simulink model "DDCU_wxt_v02_forA_OpenLoop"  (R2014a)
settings: Solver=FixedStepDiscrete  StartTime=0.0  StopTime=16  FixedStep=0.05  RelTol=1e-3
InitFcn:
  | Veh_Par_wxt
values from neighbouring files (symbols this model uses):
  ag_thr = 0.4*g    (= 3.924)    [Veh_Par_wxt.m]
  B = 2.25    [Veh_Par_wxt.m]
  bra_pre_em = 12    [Veh_Par_wxt.m]
  bra_pre_gz2 = 12/3    (= 4)    [Veh_Par_wxt.m]
  bra_pre_gz34 = 12/3    (= 4)    [Veh_Par_wxt.m]
  bra_pre_yd = 12/2    (= 6)    [Veh_Par_wxt.m]
  brakepre_dem_data = [0 1 2 3 4 5 6 7 8 9 10 11 12]    [Veh_Par_wxt.m]
  brakeTrq_dem_data = [0 218.198 436.396 654.594 872.792 1090.99 1309.188 1527.386 1745.584 1963.782 2181.98 2400.178 2618.376]    [Veh_Par_wxt.m]
  bratrq_max = 4*2618.376    (= 10473.504)    [Veh_Par_wxt.m]
  eff_tran = 0.75    [Veh_Par_wxt.m]
  G = Mass*g    (= 36297)    [Veh_Par_wxt.m]
  kd1 = 1    [Veh_Par_wxt.m]
  kd2 = 1    [Veh_Par_wxt.m]
  kd3 = 1    [Veh_Par_wxt.m]
  ki1 = 1    [Veh_Par_wxt.m]
  ki2 = 1    [Veh_Par_wxt.m]
  ki3 = 1    [Veh_Par_wxt.m]
  kp1 = 1    [Veh_Par_wxt.m]
  kp2 = 1    [Veh_Par_wxt.m]
  kp3 = 1    [Veh_Par_wxt.m]
  L = 3.12    [Veh_Par_wxt.m]
  premax = 12    [Veh_Par_wxt.m]
  Radius = 0.20    (= 0.2)    [Veh_Par_wxt.m]
  s_opt_yi_add = 0.05    [Veh_Par_wxt.m]
  s_opt_zhuan_add = 0.05    [Veh_Par_wxt.m]
  spd_map_mot = [0 100 200 300 360 400 500 600 700 800 900]*tras_ratio    [Veh_Par_wxt.m]
  spdmax = 900*tras_ratio    (= 5580)    [Veh_Par_wxt.m]
  speed_thr_park = 5/3.6/Radius*30/pi    (= 66.3145596216)    [Veh_Par_wxt.m]
  tras_ratio = 6.2    [Veh_Par_wxt.m]
  trq_map_mot = [1200 1200 1200 1200 1200 1080 864 720 617 540 480]/tras_ratio    [Veh_Par_wxt.m]
  trqmax = 80    [Veh_Par_wxt.m]
  v_thr1_b = 5    [Veh_Par_wxt.m]
  v_thr2_b = 20    [Veh_Par_wxt.m]
  v_thr_park = 5    [Veh_Par_wxt.m]
undefined symbols (not defined in the file or in its folder): DiscIntNeverNeededParam, sigbuilder_block
libraries: simulink x169, ec5744lib x9
(part 5 of 13)

== system DDCU_wxt_v02_forA_OpenLoop/OutputSignalProcess/VCU_MCU2_replace/M4Mode ==
  M4Mode : Inport
  Constant{1..4,6..8} (7 alike) : Constant  Value=0  OutDataTypeStr=uint8
  M4ModeRon : Rounding  Operator=round
  M4Mode_1sat : Saturate  UpperLimit=3  LowerLimit=0
  M4Mode_Convert : DataTypeConversion  OutDataTypeStr=uint8
  M4Mode_Convert1 : DataTypeConversion  OutDataTypeStr=uint32
  M4Mode_D : Product  Inputs=*/
  M4Mode_F : Constant  OutDataTypeStr=single
  M4Mode_L : simulink/Logic and Bit Operations/Bitwise Operator  logicop=AND  UseBitMask=on  BitMask=3  BitMaskRealWorld=Stored Integer
  M4Mode_O : Constant  Value=0  OutDataTypeStr=single
  M4Mode_S : ArithShift
  M4Mode_sat : Saturate  UpperLimit=3  LowerLimit=0
  M4Mode_st : Sum  Inputs=+-
  output1 : Outport
  output2 : Outport  Port=2
  output3 : Outport  Port=3
  output4 : Outport  Port=4
  output5 : Outport  Port=5
  output6 : Outport  Port=6
  output7 : Outport  Port=7
  output8 : Outport  Port=8
  wires:
  M4Mode/1 -> M4Mode_sat/1
  M4Mode_sat/1 -> M4Mode_st/1
  M4Mode_O/1 -> M4Mode_st/2
  M4Mode_st/1 -> M4Mode_D/1
  M4Mode_F/1 -> M4Mode_D/2
  M4Mode_D/1 -> M4ModeRon/1
  M4ModeRon/1 -> M4Mode_S/1
  M4Mode_S/1 -> M4Mode_1sat/1
  M4Mode_1sat/1 -> M4Mode_Convert1/1
  M4Mode_Convert1/1 -> M4Mode_L/1
  M4Mode_L/1 -> M4Mode_Convert/1
  M4Mode_Convert/1 -> output5/1
  Constant1/1 -> output1/1
  Constant2/1 -> output2/1
  Constant3/1 -> output3/1
  Constant4/1 -> output4/1
  Constant6/1 -> output6/1
  Constant7/1 -> output7/1
  Constant8/1 -> output8/1

== system DDCU_wxt_v02_forA_OpenLoop/OutputSignalProcess/VCU_MCU2_replace/M4SpeedLimit ==
  M4SpeedLimit : Inport
  Constant{1..6} (6 alike) : Constant  Value=0  OutDataTypeStr=uint8
  M4SpeedLimitBitCov : DataTypeConversion  OutDataTypeStr=uint8
  M4SpeedLimitCOV : DataTypeConversion  OutDataTypeStr=uint8
  M4SpeedLimitRon : Rounding  Operator=round
  M4SpeedLimit_1sat : Saturate  UpperLimit=4095  LowerLimit=0
  M4SpeedLimit_And : simulink/Logic and Bit Operations/Bitwise Operator  logicop=AND  UseBitMask=off  NumInputPorts=2  BitMask=bin2dec('11011001')  BitMaskRealWorld=Stored Integer
  M4SpeedLimit_And_C : Constant  Value=255  OutDataTypeStr=uint32
  M4SpeedLimit_Convert : DataTypeConversion  OutDataTypeStr=uint32
  M4SpeedLimit_D : Product  Inputs=*/
  M4SpeedLimit_D1 : Product  Inputs=*/
  M4SpeedLimit_F : Constant  Value=5  OutDataTypeStr=single
  M4SpeedLimit_L : simulink/Logic and Bit Operations/Bitwise Operator  logicop=AND  UseBitMask=on  BitMask=4095  BitMaskRealWorld=Stored Integer
  M4SpeedLimit_O : Constant  Value=0  OutDataTypeStr=single
  M4SpeedLimit_S : ArithShift
  M4SpeedLimit_sat : Saturate  UpperLimit=20475  LowerLimit=0
  M4SpeedLimit_st : Sum  Inputs=+-
  M4SpeedLimitoutput8_C : Constant  Value=256
  output1 : Outport
  output2 : Outport  Port=2
  output3 : Outport  Port=3
  output4 : Outport  Port=4
  output5 : Outport  Port=5
  output6 : Outport  Port=6
  output7 : Outport  Port=7
  output8 : Outport  Port=8
  wires:
  M4SpeedLimit/1 -> M4SpeedLimit_sat/1
  M4SpeedLimit_sat/1 -> M4SpeedLimit_st/1
  M4SpeedLimit_O/1 -> M4SpeedLimit_st/2
  M4SpeedLimit_st/1 -> M4SpeedLimit_D/1
  M4SpeedLimit_F/1 -> M4SpeedLimit_D/2
  M4SpeedLimit_D/1 -> M4SpeedLimitRon/1
  M4SpeedLimitRon/1 -> M4SpeedLimit_S/1
  M4SpeedLimit_S/1 -> M4SpeedLimit_1sat/1
  M4SpeedLimit_1sat/1 -> M4SpeedLimit_Convert/1
  M4SpeedLimit_Convert/1 -> M4SpeedLimit_L/1
  M4SpeedLimit_L/1 -> M4SpeedLimit_D1/1, M4SpeedLimit_And/1
  M4SpeedLimitoutput8_C/1 -> M4SpeedLimit_D1/2
  M4SpeedLimit_D1/1 -> M4SpeedLimitCOV/1
  M4SpeedLimitCOV/1 -> output8/1
  M4SpeedLimit_And_C/1 -> M4SpeedLimit_And/2
  M4SpeedLimit_And/1 -> M4SpeedLimitBitCov/1
  M4SpeedLimitBitCov/1 -> output7/1
  Constant1/1 -> output1/1
  Constant2/1 -> output2/1
  Constant3/1 -> output3/1
  Constant4/1 -> output4/1
  Constant5/1 -> output5/1
  Constant6/1 -> output6/1

== system DDCU_wxt_v02_forA_OpenLoop/OutputSignalProcess/VCU_MCU2_replace/M4SpeedSet ==
  M4SpeedSet : Inport
  Constant{1..4,7..8} (6 alike) : Constant  Value=0  OutDataTypeStr=uint8
  M4SpeedSetBitCov : DataTypeConversion  OutDataTypeStr=uint8
  M4SpeedSetCOV : DataTypeConversion  OutDataTypeStr=uint8
  M4SpeedSetRon : Rounding  Operator=round
  M4SpeedSet_1sat : Saturate  UpperLimit=65520  LowerLimit=0
  M4SpeedSet_And : simulink/Logic and Bit Operations/Bitwise Operator  logicop=AND  UseBitMask=off  NumInputPorts=2  BitMask=bin2dec('11011001')  BitMaskRealWorld=Stored Integer
  M4SpeedSet_And_C : Constant  Value=255  OutDataTypeStr=uint32
  M4SpeedSet_Convert : DataTypeConversion  OutDataTypeStr=uint32
  M4SpeedSet_D : Product  Inputs=*/
  M4SpeedSet_D1 : Product  Inputs=*/
  M4SpeedSet_F : Constant  Value=5  OutDataTypeStr=single
  M4SpeedSet_L : simulink/Logic and Bit Operations/Bitwise Operator  logicop=AND  UseBitMask=on  BitMask=65520  BitMaskRealWorld=Stored Integer
  M4SpeedSet_O : Constant  Value=-5000  OutDataTypeStr=single
  M4SpeedSet_S : ArithShift  BitShiftNumber=-4
  M4SpeedSet_sat : Saturate  UpperLimit=15475  LowerLimit=-5000
  M4SpeedSet_st : Sum  Inputs=+-
  M4SpeedSetoutput6_C : Constant  Value=256
  output1 : Outport
  output2 : Outport  Port=2
  output3 : Outport  Port=3
  output4 : Outport  Port=4
  output5 : Outport  Port=5
  output6 : Outport  Port=6
  output7 : Outport  Port=7
  output8 : Outport  Port=8
  wires:
  M4SpeedSet/1 -> M4SpeedSet_sat/1
  M4SpeedSet_sat/1 -> M4SpeedSet_st/1
  M4SpeedSet_O/1 -> M4SpeedSet_st/2
  M4SpeedSet_st/1 -> M4SpeedSet_D/1
  M4SpeedSet_F/1 -> M4SpeedSet_D/2
  M4SpeedSet_D/1 -> M4SpeedSetRon/1
  M4SpeedSetRon/1 -> M4SpeedSet_S/1
  M4SpeedSet_S/1 -> M4SpeedSet_1sat/1
  M4SpeedSet_1sat/1 -> M4SpeedSet_Convert/1
  M4SpeedSet_Convert/1 -> M4SpeedSet_L/1
  M4SpeedSet_L/1 -> M4SpeedSet_D1/1, M4SpeedSet_And/1
  M4SpeedSetoutput6_C/1 -> M4SpeedSet_D1/2
  M4SpeedSet_D1/1 -> M4SpeedSetCOV/1
  M4SpeedSetCOV/1 -> output6/1
  M4SpeedSet_And_C/1 -> M4SpeedSet_And/2
  M4SpeedSet_And/1 -> M4SpeedSetBitCov/1
  M4SpeedSetBitCov/1 -> output5/1
  Constant1/1 -> output1/1
  Constant2/1 -> output2/1
  Constant3/1 -> output3/1
  Constant4/1 -> output4/1
  Constant7/1 -> output7/1
  Constant8/1 -> output8/1

== system DDCU_wxt_v02_forA_OpenLoop/OutputSignalProcess/VCU_MCU2_replace/MCU2HeartBeat ==
  MCU2HeartBeat : Inport
  Constant{1..7} (7 alike) : Constant  Value=0  OutDataTypeStr=uint8
  MCU2HeartBeatRon : Rounding  Operator=round
  MCU2HeartBeat_1sat : Saturate  UpperLimit=240  LowerLimit=0
  MCU2HeartBeat_Convert : DataTypeConversion  OutDataTypeStr=uint8
  MCU2HeartBeat_Convert1 : DataTypeConversion  OutDataTypeStr=uint32
  MCU2HeartBeat_D : Product  Inputs=*/
  MCU2HeartBeat_F : Constant  OutDataTypeStr=single
  MCU2HeartBeat_L : simulink/Logic and Bit Operations/Bitwise Operator  logicop=AND  UseBitMask=on  BitMask=240  BitMaskRealWorld=Stored Integer
  MCU2HeartBeat_O : Constant  Value=0  OutDataTypeStr=single
  MCU2HeartBeat_S : ArithShift  BitShiftNumber=-4
  MCU2HeartBeat_sat : Saturate  UpperLimit=15  LowerLimit=0
  MCU2HeartBeat_st : Sum  Inputs=+-
  output1 : Outport
  output2 : Outport  Port=2
  output3 : Outport  Port=3
  output4 : Outport  Port=4
  output5 : Outport  Port=5
  output6 : Outport  Port=6
  output7 : Outport  Port=7
  output8 : Outport  Port=8
  wires:
  MCU2HeartBeat/1 -> MCU2HeartBeat_sat/1
  MCU2HeartBeat_sat/1 -> MCU2HeartBeat_st/1
  MCU2HeartBeat_O/1 -> MCU2HeartBeat_st/2
  MCU2HeartBeat_st/1 -> MCU2HeartBeat_D/1
  MCU2HeartBeat_F/1 -> MCU2HeartBeat_D/2
  MCU2HeartBeat_D/1 -> MCU2HeartBeatRon/1
  MCU2HeartBeatRon/1 -> MCU2HeartBeat_S/1
  MCU2HeartBeat_S/1 -> MCU2HeartBeat_1sat/1
  MCU2HeartBeat_1sat/1 -> MCU2HeartBeat_Convert1/1
  MCU2HeartBeat_Convert1/1 -> MCU2HeartBeat_L/1
  MCU2HeartBeat_L/1 -> MCU2HeartBeat_Convert/1
  MCU2HeartBeat_Convert/1 -> output8/1
  Constant1/1 -> output1/1
  Constant2/1 -> output2/1
  Constant3/1 -> output3/1
  Constant4/1 -> output4/1
  Constant5/1 -> output5/1
  Constant6/1 -> output6/1
  Constant7/1 -> output7/1

== system DDCU_wxt_v02_forA_OpenLoop/OutputSignalProcess/VCU_Park/ParkEnable ==
  ParkEnable : Inport
  Constant{2..8} (7 alike) : Constant  Value=0  OutDataTypeStr=uint8
  ParkEnableRon : Rounding  Operator=round
  ParkEnable_1sat : Saturate  UpperLimit=1  LowerLimit=0
  ParkEnable_Convert : DataTypeConversion  OutDataTypeStr=uint8
  ParkEnable_Convert1 : DataTypeConversion  OutDataTypeStr=uint32
  ParkEnable_D : Product  Inputs=*/
  ParkEnable_F : Constant  OutDataTypeStr=single
  ParkEnable_L : simulink/Logic and Bit Operations/Bitwise Operator  logicop=AND  UseBitMask=on  BitMask=1  BitMaskRealWorld=Stored Integer
  ParkEnable_O : Constant  Value=0  OutDataTypeStr=single
  ParkEnable_S : ArithShift
  ParkEnable_sat : Saturate  UpperLimit=1  LowerLimit=0
  ParkEnable_st : Sum  Inputs=+-
  output1 : Outport
  output2 : Outport  Port=2
  output3 : Outport  Port=3
  output4 : Outport  Port=4
  output5 : Outport  Port=5
  output6 : Outport  Port=6
  output7 : Outport  Port=7
  output8 : Outport  Port=8
  wires:
  ParkEnable/1 -> ParkEnable_sat/1
  ParkEnable_sat/1 -> ParkEnable_st/1
  ParkEnable_O/1 -> ParkEnable_st/2
  ParkEnable_st/1 -> ParkEnable_D/1
  ParkEnable_F/1 -> ParkEnable_D/2
  ParkEnable_D/1 -> ParkEnableRon/1
  ParkEnableRon/1 -> ParkEnable_S/1
  ParkEnable_S/1 -> ParkEnable_1sat/1
  ParkEnable_1sat/1 -> ParkEnable_Convert1/1
  ParkEnable_Convert1/1 -> ParkEnable_L/1
  ParkEnable_L/1 -> ParkEnable_Convert/1
  ParkEnable_Convert/1 -> output1/1
  Constant2/1 -> output2/1
  Constant3/1 -> output3/1
  Constant4/1 -> output4/1
  Constant5/1 -> output5/1
  Constant6/1 -> output6/1
  Constant7/1 -> output7/1
  Constant8/1 -> output8/1

== system DDCU_wxt_v02_forA_OpenLoop/Data_Input/HCU1_VCU/HCU1_VCU/acc_Sub ==
  In1 : Inport
  Out1 : Outport
  wires:
  In1/1 -> Out1/1

== system DDCU_wxt_v02_forA_OpenLoop/Data_Input/HCU1_VCU/HCU1_VCU/break_Sub ==
  In1 : Inport
  Out1 : Outport
  wires:
  In1/1 -> Out1/1

== system DDCU_wxt_v02_forA_OpenLoop/Data_Input/HCU1_VCU/HCU1_VCU/pwr_limit_Sub ==
  In1 : Inport
  Out1 : Outport
  wires:
  In1/1 -> Out1/1

== system DDCU_wxt_v02_forA_OpenLoop/Data_Input/HCU1_VCU/HCU1_VCU/real_velocity_Sub ==
  In1 : Inport
  Out1 : Outport
  wires:
  In1/1 -> Out1/1

== system DDCU_wxt_v02_forA_OpenLoop/Data_Input/HCU1_VCU/HCU1_VCU/turn_Sub ==
  In1 : Inport
  Out1 : Outport
  wires:
  In1/1 -> Out1/1

== system DDCU_wxt_v02_forA_OpenLoop/Data_Input/HCU1_VCU1/MUC1_VCU1/spd_mot_lf_Sub ==
  In1 : Inport
  Out1 : Outport
  wires:
  In1/1 -> Out1/1

== system DDCU_wxt_v02_forA_OpenLoop/Data_Input/HCU1_VCU1/MUC1_VCU1/spd_mot_lr_Sub ==
  In1 : Inport
  Out1 : Outport
  wires:
  In1/1 -> Out1/1

== system DDCU_wxt_v02_forA_OpenLoop/Data_Input/HCU1_VCU1/MUC1_VCU1/spd_mot_rf_Sub ==
  In1 : Inport
  Out1 : Outport
  wires:
  In1/1 -> Out1/1

== system DDCU_wxt_v02_forA_OpenLoop/Data_Input/HCU1_VCU1/MUC1_VCU1/spd_mot_rr_Sub ==
  In1 : Inport
  Out1 : Outport
  wires:
  In1/1 -> Out1/1

== system DDCU_wxt_v02_forA_OpenLoop/Data_Input/HCU2_VCU/HCU2_VCU/daodang_Sub ==
  In1 : Inport
  Out1 : Outport
  wires:
  In1/1 -> Out1/1

== system DDCU_wxt_v02_forA_OpenLoop/Data_Input/HCU2_VCU/HCU2_VCU/kongdang_Sub ==
  In1 : Inport
  Out1 : Outport
  wires:
  In1/1 -> Out1/1

== system DDCU_wxt_v02_forA_OpenLoop/Data_Input/HCU2_VCU/HCU2_VCU/qianjin_Sub ==
  In1 : Inport
  Out1 : Outport
  wires:
  In1/1 -> Out1/1

== system DDCU_wxt_v02_forA_OpenLoop/Data_Input/HCU2_VCU/HCU2_VCU/zhongxinzhuanxiang_Sub ==
  In1 : Inport
  Out1 : Outport
  wires:
  In1/1 -> Out1/1

== system DDCU_wxt_v02_forA_OpenLoop/Data_Input/HCU2_VCU/HCU2_VCU/zhuche_Sub ==
  In1 : Inport
  Out1 : Outport
  wires:
  In1/1 -> Out1/1

== system DDCU_wxt_v02_forA_OpenLoop/MainControl/mode_control/Park/park ==
  Signals : Inport
  1-D Lookup Table : Lookup_n-D  NumberOfTableDimensions=1  BreakpointsForDimension1=brakeTrq_dem_data  Table=brakepre_dem_data  InternalRulePriority=Speed  RndMeth=Simplest  InputSameDT=on
  1-D Lookup Table1 : Lookup_n-D  NumberOfTableDimensions=1  BreakpointsForDimension1=brakeTrq_dem_data  Table=brakepre_dem_data  InternalRulePriority=Speed  RndMeth=Simplest  InputSameDT=on
  Bus Selector : BusSelector  OutputSignals=YaoKong.brake_dem
  Constant : Constant  Value=bratrq_max
  Gain : Gain  Gain=1/2
  Gain1 : Gain  Gain=1/100
  Gain2 : Gain  Gain=1/2
  Gain3 : Gain  Gain=1/2
  HeartBeat : MATLAB Function  TreatAsAtomicUnit=on
  HeartBeat1 : MATLAB Function  TreatAsAtomicUnit=on
  Memory : Memory  InheritSampleTime=on
  Memory1 : Memory  InheritSampleTime=on
  Mux : Mux  Inputs=8
  Mux1 : Mux  Inputs=8
  Mux2 : Mux  Inputs=7
  Mux3 : Mux  Inputs=7
  Product : Product
  Saturation1 : Saturate  UpperLimit=premax  LowerLimit=0
  Saturation4 : Saturate  UpperLimit=premax  LowerLimit=0
  SpdLim_dem{,1..3} (4 alike) : Constant  Value=spdmax
  SpdSet_dem : Constant  Value=0
  SpdSet_dem1 : Constant
  SpdSet_dem2 : Constant
  SpdSet_dem3 : Constant
  TrqLim_dem{,1..3} (4 alike) : Constant
  TrqSet_dem{,1..3} (4 alike) : Constant  Value=0
  mot_drive : Constant
  mot_drive1 : Constant  Value=2
  mot_drive2 : Constant
  mot_drive3 : Constant  Value=2
  mot_enable{,1..3} (4 alike) : Constant  Value=2
  mot_mode{,1..3} (4 alike) : Constant
  mot_lf : Outport
  mot_lr : Outport  Port=2
  mot_rf : Outport  Port=3
  mot_rr : Outport  Port=4
  bra_pre_l : Outport  Port=5
  bra_pre_r : Outport  Port=6
  wires:
  mot_drive/1 -> Mux/3
  mot_mode/1 -> Mux/2
  TrqSet_dem/1 -> Mux/4
  mot_enable/1 -> Mux/1
  SpdSet_dem/1 -> Mux/5
  Mux/1 -> mot_lf/1
  Signals/1 -> Bus Selector/1
  1-D Lookup Table/1 -> Saturation4/1
  TrqLim_dem/1 -> Mux/6
  HeartBeat/1(life) -> Mux/8, Memory/1
  Memory/1 -> HeartBeat/1(life_pre)
  SpdLim_dem/1 -> Mux/7
  mot_drive1/1 -> Mux2/3
  mot_mode2/1 -> Mux2/2
  TrqSet_dem1/1 -> Mux2/4
  mot_enable2/1 -> Mux2/1
  SpdSet_dem1/1 -> Mux2/5
  Mux2/1 -> mot_rf/1
  TrqLim_dem1/1 -> Mux2/6
  SpdLim_dem1/1 -> Mux2/7
  mot_drive2/1 -> Mux1/3
  mot_mode1/1 -> Mux1/2
  TrqSet_dem2/1 -> Mux1/4
  mot_enable1/1 -> Mux1/1
  SpdSet_dem2/1 -> Mux1/5
  Mux1/1 -> mot_lr/1
  TrqLim_dem2/1 -> Mux1/6
  HeartBeat1/1(life) -> Mux1/8, Memory1/1
  Memory1/1 -> HeartBeat1/1(life_pre)
  SpdLim_dem2/1 -> Mux1/7
  mot_drive3/1 -> Mux3/3
  mot_mode3/1 -> Mux3/2
  TrqSet_dem3/1 -> Mux3/4
  mot_enable3/1 -> Mux3/1
  SpdSet_dem3/1 -> Mux3/5
  Mux3/1 -> mot_rr/1
  TrqLim_dem3/1 -> Mux3/6
  SpdLim_dem3/1 -> Mux3/7
  Constant/1 -> Product/1
  Bus Selector/1 -> Gain1/1  "<brake_dem>"
  Product/1 -> Gain/1
  Gain/1 -> Gain3/1, Gain2/1
  Gain1/1 -> Product/2
  Gain2/1 -> 1-D Lookup Table/1
  Gain3/1 -> 1-D Lookup Table1/1
  1-D Lookup Table1/1 -> Saturation1/1
  Saturation4/1 -> bra_pre_l/1
  Saturation1/1 -> bra_pre_r/1

== system DDCU_wxt_v02_forA_OpenLoop/MainControl/mode_control/backward/backward ==
  Signals : Inport
  Brake : Subsystem  TreatAsAtomicUnit=on
  Bus Selector : BusSelector  OutputSignals=YaoKong.acc_dem,YaoKong.brake_dem,YaoKong.HAC
  Constant : Constant  Value=0.15
  Drive : Subsystem  TreatAsAtomicUnit=on
  MATLAB Function : MATLAB Function  TreatAsAtomicUnit=on
  Multiport Switch : MultiPortSwitch  DataPortOrder=Zero-based contiguous  Inputs=2
  Switch Case1 : SwitchCase  CaseConditions={0,1}  ShowDefaultCase=off
  backward_dem : Outport
  wires:
  Constant/1 -> Brake/2(s_opt_yi)
  Brake/1(backward_dem) -> Multiport Switch/3
  Drive/1(backward_dem) -> Multiport Switch/2
  MATLAB Function/1(y) -> Switch Case1/1, Multiport Switch/1
  Switch Case1/2 -> Brake/Action
  Switch Case1/1 -> Drive/Action
  Multiport Switch/1 -> backward_dem/1
  Signals/1 -> Bus Selector/1, Drive/1(Signals), Brake/1(Signals)
  Bus Selector/1 -> MATLAB Function/1(acc_dem)  "<acc_dem>"
  Bus Selector/2 -> MATLAB Function/2(brake_dem)  "<brake_dem>"
  Bus Selector/3 -> MATLAB Function/3(HAC)  "<HAC>"

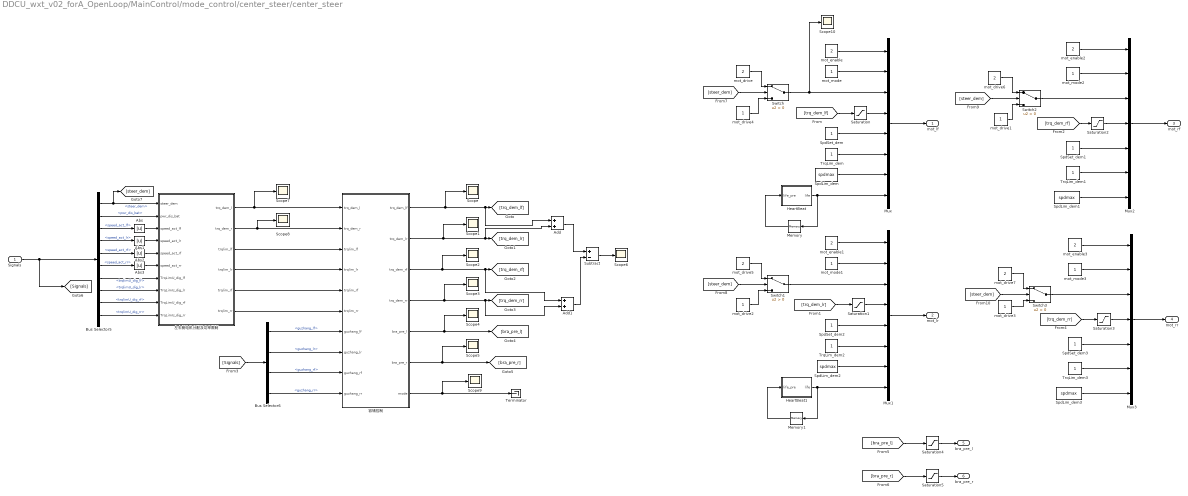
== system DDCU_wxt_v02_forA_OpenLoop/MainControl/mode_control/center_steer/center_steer ==
  Signals : Inport
  Abs{,1..3} (4 alike) : Abs
  Add : Sum
  Add1 : Sum
  Bus Selector5 : BusSelector  OutputSignals=YaoKong.steer_dem,Bat.pwr_dis_bat,DriveMotor.speed_act_lf,DriveMotor.speed_act_lr,DriveMotor.speed_act_rf,DriveMotor.speed_act_rr,DriveMotor.trqlimU_dig_lf,DriveMotor.trqlimU_dig_lr,DriveMotor.trqlimU_dig_rf,DriveMotor.trqlimU_dig_rr
  Bus Selector6 : BusSelector  OutputSignals=DriveMotor.guzhang_lf,DriveMotor.guzhang_lr,DriveMotor.guzhang_rf,DriveMotor.guzhang_rr
  HeartBeat : MATLAB Function  TreatAsAtomicUnit=on
  HeartBeat1 : MATLAB Function  TreatAsAtomicUnit=on
  Memory : Memory  InheritSampleTime=on
  Memory1 : Memory  InheritSampleTime=on
  Mux : Mux  Inputs=8
  Mux1 : Mux  Inputs=8
  Mux2 : Mux  Inputs=7
  Mux3 : Mux  Inputs=7
  Saturation{,1..3} (4 alike) : Saturate  UpperLimit=trqmax  LowerLimit=0
  Saturation4 : Saturate  UpperLimit=premax  LowerLimit=0
  Saturation5 : Saturate  UpperLimit=premax  LowerLimit=0
  Scope{,1..10} (11 alike) : Scope
      Scope settings: SaveName=ScopeData47
      Scope1 settings: SaveName=ScopeData48
      Scope10 settings: SaveName=ScopeData58
      Scope2 settings: SaveName=ScopeData49
      Scope3 settings: SaveName=ScopeData50
      Scope4 settings: SaveName=ScopeData51
      Scope5 settings: SaveName=ScopeData52
      Scope6 settings: SaveName=ScopeData54
      Scope7 settings: SaveName=ScopeData55
      Scope8 settings: SaveName=ScopeData56
      Scope9 settings: SaveName=ScopeData57
  SpdLim_dem{,1..3} (4 alike) : Constant  Value=spdmax
  SpdSet_dem{,1..3} (4 alike) : Constant
  Subtract : Sum  Inputs=+-
  Switch{,1..3} (4 alike) : Switch  Criteria=u2 > Threshold
  Terminator : Terminator
  TrqLim_dem{,1..3} (4 alike) : Constant
  mot_drive{,5..7} (4 alike) : Constant  Value=2
  mot_drive{1..4} (4 alike) : Constant
  mot_enable{,1..3} (4 alike) : Constant  Value=2
  mot_mode{,1..3} (4 alike) : Constant
  容错控制 : Subsystem
  左右侧电机分配及功率限制 : Subsystem
  mot_lf : Outport
  mot_lr : Outport  Port=2
  mot_rf : Outport  Port=3
  mot_rr : Outport  Port=4
  bra_pre_l : Outport  Port=5
  bra_pre_r : Outport  Port=6
  wires:
  Signals/1 -> [Signals], Bus Selector5/1
  Bus Selector5/2 -> 左右侧电机分配及功率限制/2(pwr_dis_bat)  "<pwr_dis_bat>"
  Bus Selector5/3 -> Abs/1  "<speed_act_lf>"
  Bus Selector5/4 -> Abs1/1  "<speed_act_lr>"
  Bus Selector5/5 -> Abs2/1  "<speed_act_rf>"
  Bus Selector5/6 -> Abs3/1  "<speed_act_rr>"
  Bus Selector5/10 -> 左右侧电机分配及功率限制/10(TrqLimU_dig_rr)  "<trqlimU_dig_rr>"
  Bus Selector5/9 -> 左右侧电机分配及功率限制/9(TrqLimU_dig_rf)  "<trqlimU_dig_rf>"
  Bus Selector5/7 -> 左右侧电机分配及功率限制/7(TrqLimU_dig_lf)  "<trqlimU_dig_lf>"
  Bus Selector5/8 -> 左右侧电机分配及功率限制/8(TrqLimU_dig_lr)  "<trqlimU_dig_lr>"
  [Signals] -> Bus Selector6/1
  左右侧电机分配及功率限制/2(trq_dem_r) -> Scope8/1, 容错控制/2(trq_dem_r)
  左右侧电机分配及功率限制/1(trq_dem_l) -> Scope7/1, 容错控制/1(trq_dem_l)
  Bus Selector6/4 -> 容错控制/10(guzhang_rr)  "<guzhang_rr>"
  Bus Selector6/3 -> 容错控制/9(guzhang_rf)  "<guzhang_rf>"
  Bus Selector6/2 -> 容错控制/8(guzhang_lr)  "<guzhang_lr>"
  Bus Selector6/1 -> 容错控制/7(guzhang_lf)  "<guzhang_lf>"
  左右侧电机分配及功率限制/5(trqlim_rf) -> 容错控制/5(trqlim_rf)
  左右侧电机分配及功率限制/4(trqlim_lr) -> 容错控制/4(trqlim_lr)
  左右侧电机分配及功率限制/6(trqlim_rr) -> 容错控制/6(trqlim_rr)
  左右侧电机分配及功率限制/3(trqlim_lf) -> 容错控制/3(trqlim_lf)
  Bus Selector5/1 -> 左右侧电机分配及功率限制/1(steer_dem), [steer_dem]  "<steer_dem>"
  容错控制/1(trq_dem_lf) -> Scope/1, Add/1, [trq_dem_lf]
  容错控制/3(trq_dem_rf) -> Scope2/1, Add1/1, [trq_dem_rf]
  容错控制/4(trq_dem_rr) -> Scope3/1, Add1/2, [trq_dem_rr]
  容错控制/5(bra_pre_l) -> Scope4/1, [bra_pre_l]
  容错控制/6(bra_pre_r) -> Scope5/1, [bra_pre_r]
  容错控制/2(trq_dem_lr) -> Scope1/1, Add/2, [trq_dem_lr]
  Switch/1 -> Scope10/1, Mux/3
  mot_mode/1 -> Mux/2
  [trq_dem_lf] -> Saturation/1
  mot_enable/1 -> Mux/1
  SpdSet_dem/1 -> Mux/5
  Mux/1 -> mot_lf/1
  TrqLim_dem/1 -> Mux/6
  HeartBeat/1(life) -> Mux/8, Memory/1
  Memory/1 -> HeartBeat/1(life_pre)
  SpdLim_dem/1 -> Mux/7
  Switch2/1 -> Mux2/3
  mot_mode2/1 -> Mux2/2
  [trq_dem_rf] -> Saturation2/1
  mot_enable2/1 -> Mux2/1
  SpdSet_dem1/1 -> Mux2/5
  Mux2/1 -> mot_rf/1
  TrqLim_dem1/1 -> Mux2/6
  SpdLim_dem1/1 -> Mux2/7
  Switch1/1 -> Mux1/3
  mot_mode1/1 -> Mux1/2
  [trq_dem_lr] -> Saturation1/1
  mot_enable1/1 -> Mux1/1
  SpdSet_dem2/1 -> Mux1/5
  Mux1/1 -> mot_lr/1
  TrqLim_dem2/1 -> Mux1/6
  HeartBeat1/1(life) -> Mux1/8, Memory1/1
  Memory1/1 -> HeartBeat1/1(life_pre)
  SpdLim_dem2/1 -> Mux1/7
  Switch3/1 -> Mux3/3
  mot_mode3/1 -> Mux3/2
  [trq_dem_rr] -> Saturation3/1
  mot_enable3/1 -> Mux3/1
  SpdSet_dem3/1 -> Mux3/5
  Mux3/1 -> mot_rr/1
  TrqLim_dem3/1 -> Mux3/6
  SpdLim_dem3/1 -> Mux3/7
  [bra_pre_l] -> Saturation4/1
  [bra_pre_r] -> Saturation5/1
  Saturation/1 -> Mux/4
  Saturation1/1 -> Mux1/4
  Saturation2/1 -> Mux2/4
  Saturation3/1 -> Mux3/4
  Saturation4/1 -> bra_pre_l/1
  Saturation5/1 -> bra_pre_r/1
  Add/1 -> Subtract/1
  Add1/1 -> Subtract/2
  Subtract/1 -> Scope6/1
  容错控制/7(mode) -> Terminator/1, Scope9/1
  Abs/1 -> 左右侧电机分配及功率限制/3(speed_act_lf)
  Abs1/1 -> 左右侧电机分配及功率限制/4(speed_act_lr)
  Abs2/1 -> 左右侧电机分配及功率限制/5(speed_act_rf)
  Abs3/1 -> 左右侧电机分配及功率限制/6(speed_act_rr)
  [steer_dem] -> Switch/2
  mot_drive4/1 -> Switch/3
  mot_drive/1 -> Switch/1
  [steer_dem] -> Switch1/2
  mot_drive5/1 -> Switch1/1
  mot_drive2/1 -> Switch1/3
  [steer_dem] -> Switch2/2
  mot_drive6/1 -> Switch2/1
  mot_drive1/1 -> Switch2/3
  [steer_dem] -> Switch3/2
  mot_drive7/1 -> Switch3/1
  mot_drive3/1 -> Switch3/3

== system DDCU_wxt_v02_forA_OpenLoop/MainControl/mode_control/emergency_stop/emergency_stop ==
  Signals : Inport
  Bus Selector : BusSelector  OutputSignals=YaoKong.brake_dem
  Constant : Constant  Value=bra_pre_em
  HeartBeat : MATLAB Function  TreatAsAtomicUnit=on
  HeartBeat1 : MATLAB Function  TreatAsAtomicUnit=on
  Memory : Memory  InheritSampleTime=on
  Memory1 : Memory  InheritSampleTime=on
  Mux : Mux  Inputs=8
  Mux1 : Mux  Inputs=8
  Mux2 : Mux  Inputs=7
  Mux3 : Mux  Inputs=7
  Saturation1 : Saturate  UpperLimit=premax  LowerLimit=0
  Saturation4 : Saturate  UpperLimit=premax  LowerLimit=0
  SpdLim_dem{,1..3} (4 alike) : Constant  Value=spdmax
  SpdSet_dem{,1..3} (4 alike) : Constant
  Terminator : Terminator
  TrqLim_dem{,1..3} (4 alike) : Constant
  TrqSet_dem{,1..3} (4 alike) : Constant  Value=0
  mot_drive : Constant
  mot_drive1 : Constant  Value=2
  mot_drive2 : Constant
  mot_drive3 : Constant  Value=2
  mot_enable{,1..3} (4 alike) : Constant  Value=2
  mot_mode{,1..3} (4 alike) : Constant
  mot_lf : Outport
  mot_lr : Outport  Port=2
  mot_rf : Outport  Port=3
  mot_rr : Outport  Port=4
  bra_pre_l : Outport  Port=5
  bra_pre_r : Outport  Port=6
  wires:
  mot_drive/1 -> Mux/3
  mot_mode/1 -> Mux/2
  TrqSet_dem/1 -> Mux/4
  mot_enable/1 -> Mux/1
  SpdSet_dem/1 -> Mux/5
  Mux/1 -> mot_lf/1
  Signals/1 -> Bus Selector/1
  Bus Selector/1 -> Terminator/1  "<brake_dem>"
  TrqLim_dem/1 -> Mux/6
  HeartBeat/1(life) -> Mux/8, Memory/1
  Memory/1 -> HeartBeat/1(life_pre)
  SpdLim_dem/1 -> Mux/7
  mot_drive1/1 -> Mux2/3
  mot_mode2/1 -> Mux2/2
  TrqSet_dem1/1 -> Mux2/4
  mot_enable2/1 -> Mux2/1
  SpdSet_dem1/1 -> Mux2/5
  Mux2/1 -> mot_rf/1
  TrqLim_dem1/1 -> Mux2/6
  SpdLim_dem1/1 -> Mux2/7
  mot_drive2/1 -> Mux1/3
  mot_mode1/1 -> Mux1/2
  TrqSet_dem2/1 -> Mux1/4
  mot_enable1/1 -> Mux1/1
  SpdSet_dem2/1 -> Mux1/5
  Mux1/1 -> mot_lr/1
  TrqLim_dem2/1 -> Mux1/6
  HeartBeat1/1(life) -> Mux1/8, Memory1/1
  Memory1/1 -> HeartBeat1/1(life_pre)
  SpdLim_dem2/1 -> Mux1/7
  mot_drive3/1 -> Mux3/3
  mot_mode3/1 -> Mux3/2
  TrqSet_dem3/1 -> Mux3/4
  mot_enable3/1 -> Mux3/1
  SpdSet_dem3/1 -> Mux3/5
  Mux3/1 -> mot_rr/1
  TrqLim_dem3/1 -> Mux3/6
  SpdLim_dem3/1 -> Mux3/7
  Constant/1 -> Saturation4/1, Saturation1/1
  Saturation4/1 -> bra_pre_l/1
  Saturation1/1 -> bra_pre_r/1

== system DDCU_wxt_v02_forA_OpenLoop/MainControl/mode_control/forward/forward ==
  Signals : Inport
  Brake : Subsystem  TreatAsAtomicUnit=on
  Bus Selector : BusSelector  OutputSignals=YaoKong.acc_dem,YaoKong.brake_dem,YaoKong.HAC
  Constant : Constant  Value=0.15
  Drive : Subsystem  TreatAsAtomicUnit=on
  MATLAB Function : MATLAB Function  TreatAsAtomicUnit=on
  Multiport Switch : MultiPortSwitch  DataPortOrder=Zero-based contiguous  Inputs=2
  Switch Case1 : SwitchCase  CaseConditions={0,1}  ShowDefaultCase=off
  forward_dem : Outport
  wires:
  Signals/1 -> Brake/1(Signals), Drive/1(Signals), Bus Selector/1
  Multiport Switch/1 -> forward_dem/1
  Switch Case1/1 -> Drive/Action
  Switch Case1/2 -> Brake/Action
  Bus Selector/1 -> MATLAB Function/1(acc_dem)  "<acc_dem>"
  MATLAB Function/1(y) -> Multiport Switch/1, Switch Case1/1
  Drive/1(forward_dem) -> Multiport Switch/2
  Brake/1(forward_dem) -> Multiport Switch/3
  Constant/1 -> Brake/2(s_opt_yi)
  Bus Selector/2 -> MATLAB Function/2(brake_dem)  "<brake_dem>"
  Bus Selector/3 -> MATLAB Function/3(HAC)  "<HAC>"

== matlab function DDCU_wxt_v02_forA_OpenLoop/MainControl/mode_control/forward/forward/Drive/驱动防滑控制TCS/直行TCS/直行/MATLAB Function1 ==
  data: s_act_lr input; flag_lr output; s_opt_zhuan input; s_opt_zhuan_add input; flag_lr_pre input
function flag_lr = fcn(s_act_lr,s_opt_zhuan,s_opt_zhuan_add,flag_lr_pre)
%#codegen
if s_act_lr>s_opt_zhuan+s_opt_zhuan_add
    flag_lr=1;
elseif s_act_lr<s_opt_zhuan
    flag_lr = 0;
else
    flag_lr=flag_lr_pre;
end
end

== matlab function DDCU_wxt_v02_forA_OpenLoop/MainControl/mode_control/backward/backward/Brake/HeartBeat1 ==
  data: life_pre input; life output
function life = fcn(life_pre)
%#codegen
life=life_pre+1;
if life>15
    life=0;
end
end

== matlab function DDCU_wxt_v02_forA_OpenLoop/MainControl/mode_control/backward/backward/Brake/MATLAB Function2 ==
  data: syi_act_lr input; flagyi_lr output; s_opt_yi input; s_opt_yi_add input; flagyi_lr_pre input
function flagyi_lr = fcn(syi_act_lr,s_opt_yi,s_opt_yi_add,flagyi_lr_pre)
%#codegen
if syi_act_lr>s_opt_yi+s_opt_yi_add
    flagyi_lr=1;
elseif syi_act_lr<s_opt_yi
    flagyi_lr = 0;
else
    flagyi_lr=flagyi_lr_pre;
end
end

== matlab function DDCU_wxt_v02_forA_OpenLoop/MainControl/mode_control/backward/backward/Drive/左右侧电机分配及功率限制/MATLAB Function ==
  data: trqlim_l input; trq_dem_l output; trq_dem_r output; trq_dem_l1 input; trqlim_r input; trq_dem_r1 input; delta_T_dem input
function [trq_dem_l,trq_dem_r] = fcn(trqlim_l,trq_dem_l1,trqlim_r,trq_dem_r1,delta_T_dem)
%#codegen
if trq_dem_l1==trqlim_l
    trq_dem_l=trq_dem_l1;
    trq_dem_r=trq_dem_l1+delta_T_dem;%这时候加的是负值
elseif trq_dem_r1==trqlim_r
    trq_dem_l=trq_dem_r1-delta_T_dem;
    trq_dem_r=trq_dem_r1;
    
else
    trq_dem_l=trq_dem_l1;
    trq_dem_r=trq_dem_r1;
end
% trq_dem_l=max(0,trq_dem_l);%限一下最小值，不要小于0
% trq_dem_r=max(0,trq_dem_r);
trq_dem_l=max(-trqlim_l,trq_dem_l);%小转向半径下，内侧履带是可能输出负转矩的，从地面吸收功率，给外侧，所以不能限到0，限到最大电机外特性负值
trq_dem_r=max(-trqlim_r,trq_dem_r);
end

== matlab function DDCU_wxt_v02_forA_OpenLoop/MainControl/mode_control/backward/backward/Drive/驱动防滑控制TCS/直行TCS/直行/MATLAB Function4 ==
  data: trq_dem_lf input; trq_dem_lr input; trq_dem_rf input; trq_dem_rr input; bra_pre_l input; bra_pre_r input; brakepre_dem input; flag_lf input; flag_lr input; trq_out_lf output; flag_rf input; flag_rr input; trq_out_lr output; trq_out_rf output; trq_out_rr output; trq_pid_lf input; trq_pid_lr input; trq_pid_rf input; trq_pid_rr input; brapre_out_l output; brapre_out_r output; mode output
function [trq_out_lf,trq_out_lr,trq_out_rf,trq_out_rr,brapre_out_l,brapre_out_r,mode] = fcn(trq_dem_lf,trq_dem_lr,trq_dem_rf,trq_dem_rr,bra_pre_l,bra_pre_r,brakepre_dem,flag_lf,flag_lr,flag_rf,flag_rr,trq_pid_lf,trq_pid_lr,trq_pid_rf,trq_pid_rr)
%#codegen pid模块在外面做，里面进行十六种情况的判断，先看一下效果，不能再修改。
if flag_lf==0 && flag_lr==0 && flag_rf==0 && flag_rr==0 % 0电机滑转===============================================0电机滑转
    trq_out_lf=trq_dem_lf;
    trq_out_lr=trq_dem_lr;
    trq_out_rf=trq_dem_rf;
    trq_out_rr=trq_dem_rr;
    brapre_out_l=bra_pre_l+brakepre_dem;
    brapre_out_r=bra_pre_r+brakepre_dem;
    mode=1;
elseif flag_lf==1 && flag_lr==0 &&flag_rf==0 && flag_rr==0 %左前轮滑转===================================================1电机滑转
    trq_out_lf=trq_pid_lf;
    trq_out_lr=trq_dem_lr+(trq_dem_lf-trq_out_lf);
    trq_out_rf=trq_dem_rf;
    trq_out_rr=trq_dem_rr;
    brapre_out_l=bra_pre_l+brakepre_dem;
    brapre_out_r=bra_pre_r+brakepre_dem;
    mode=2;
elseif flag_lf==0 && flag_lr==1 &&flag_rf==0 && flag_rr==0 %左后轮滑转
    trq_out_lr=trq_pid_lr;
    trq_out_lf=trq_dem_lf+(trq_dem_lr-trq_out_lr);
    trq_out_rf=trq_dem_rf;
    trq_out_rr=trq_dem_rr;
    brapre_out_l=bra_pre_l+brakepre_dem;
    brapre_out_r=bra_pre_r+brakepre_dem;
    mode=3;
elseif flag_lf==0 && flag_lr==0 &&flag_rf==1 && flag_rr==0 %右前轮滑转
    trq_out_rf=trq_pid_rf;
    trq_out_rr=trq_dem_rr+(trq_dem_rf-trq_out_rf);
    trq_out_lf=trq_dem_lf;
    trq_out_lr=trq_dem_lr;
    brapre_out_l=bra_pre_l+brakepre_dem;
    brapre_out_r=bra_pre_r+brakepre_dem;
    mode=4;
elseif flag_lf==0 && flag_lr==0 &&flag_rf==0 && flag_rr==1 %右后轮滑转
    trq_out_rr=trq_pid_rr;
    trq_out_rf=trq_dem_rf+(trq_dem_rr-trq_out_rr);
    trq_out_lf=trq_dem_lf;
    trq_out_lr=trq_dem_lr;
    brapre_out_l=bra_pre_l+brakepre_dem;
    brapre_out_r=bra_pre_r+brakepre_dem;
    mode=5;
elseif flag_lf==1 && flag_lr==1 &&flag_rf==0 && flag_rr==0 %左侧两轮滑转=====================================================================2电机滑转
    trq_out_lf=trq_pid_lf;
    trq_out_lr=trq_pid_lr;
    trq_out_rf=trq_dem_rf-(trq_dem_lf+trq_dem_lr-trq_out_lf-trq_out_lr)/2;
    trq_out_rr=trq_dem_rr-(trq_dem_lf+trq_dem_lr-trq_out_lf-trq_out_lr)/2;
    brapre_out_l=bra_pre_l+brakepre_dem;
    brapre_out_r=bra_pre_r+brakepre_dem;
    mode=6;
elseif flag_lf==0 && flag_lr==0 &&flag_rf==1 && flag_rr==1 %右侧两轮滑转
    trq_out_rf=trq_pid_rf;
    trq_out_rr=trq_pid_rr;
    trq_out_lf=trq_dem_lf-(trq_dem_rf+trq_dem_rr-trq_out_rf-trq_out_rr)/2;
    trq_out_lr=trq_dem_lr-(trq_dem_rf+trq_dem_rr-trq_out_rf-trq_out_rr)/2;
    brapre_out_l=bra_pre_l+brakepre_dem;
    brapre_out_r=bra_pre_r+brakepre_dem;
    mode=7;
elseif flag_lf==1 && flag_lr==0 &&flag_rf==1 && flag_rr==0 %前轴滑转
    trq_out_lf=trq_pid_lf;
    trq_out_lr=trq_dem_lr+(trq_dem_lf-trq_out_lf);
    trq_out_rf=trq_pid_rf;
    trq_out_rr=trq_dem_rr+(trq_dem_rf-trq_out_rf);
    brapre_out_l=bra_pre_l+brakepre_dem;
    brapre_out_r=bra_pre_r+brakepre_dem;
    mode=8;
elseif flag_lf==0 && flag_lr==1 &&flag_rf==0 && flag_rr==1 %后轴滑转
    trq_out_lr=trq_pid_lr;
    trq_out_lf=trq_dem_lf+(trq_dem_lr-trq_out_lr);
    trq_out_rr=trq_pid_rr;
    trq_out_rf=trq_dem_rf+(trq_dem_rr-trq_out_rr);
    brapre_out_l=bra_pre_l+brakepre_dem;
    brapre_out_r=bra_pre_r+brakepre_dem;
    mode=9;
elseif flag_lf==1 && flag_lr==0 &&flag_rf==0 && flag_rr==1 %左前轮和右后轮滑转
    trq_out_lf=trq_pid_lf;
    trq_out_lr=trq_dem_lr+(trq_dem_lf-trq_out_lf);
    trq_out_rr=trq_pid_rr;
    trq_out_rf=trq_dem_rf+(trq_dem_rr-trq_out_rr);
    brapre_out_l=bra_pre_l+brakepre_dem;
    brapre_out_r=bra_pre_r+brakepre_dem;
    mode=10;
elseif flag_lf==0 && flag_lr==1 &&flag_rf==1 && flag_rr==0 %左后轮和右前轮滑转
    trq_out_lr=trq_pid_lr;
    trq_out_lf=trq_dem_lf+(trq_dem_lr-trq_out_lr);
    trq_out_rf=trq_pid_rf;
    trq_out_rr=trq_dem_rr+(trq_dem_rf-trq_out_rf);
    brapre_out_l=bra_pre_l+brakepre_dem;
    brapre_out_r=bra_pre_r+brakepre_dem;
    mode=11;
elseif flag_lf==1 && flag_lr==1 &&flag_rf==1 && flag_rr==0 %右后不滑转======================================================================3电机滑转
    trq_out_lf=trq_pid_lf;
    trq_out_lr=trq_pid_lr;
    trq_out_rf=trq_pid_rf;
    trq_out_rr=trq_dem_rr+(trq_dem_rf-trq_out_rf)-(trq_dem_lf+trq_dem_lr-trq_out_lf-trq_out_lr);
    brapre_out_l=bra_pre_l+brakepre_dem;
    brapre_out_r=bra_pre_r+brakepre_dem;
    mode=12;
elseif flag_lf==1 && flag_lr==1 &&flag_rf==0 && flag_rr==1 %右前不滑转
    trq_out_lf=trq_pid_lf;
    trq_out_lr=trq_pid_lr;
    trq_out_rr=trq_pid_rr;
    trq_out_rf=trq_dem_rf+(trq_dem_rr-trq_out_rr)-(trq_dem_lf+trq_dem_lr-trq_out_lf-trq_out_lr);
    brapre_out_l=bra_pre_l+brakepre_dem;
    brapre_out_r=bra_pre_r+brakepre_dem;
    mode=13;
elseif flag_lf==1 && flag_lr==0 &&flag_rf==1 && flag_rr==1 %左后不滑转
    trq_out_rf=trq_pid_rf;
    trq_out_rr=trq_pid_rr;
    trq_out_lf=trq_pid_lf;
    trq_out_lr=trq_dem_lr+(trq_dem_lf-trq_out_lf)-(trq_dem_rf+trq_dem_rr-trq_out_rf-trq_out_rr);
    brapre_out_l=bra_pre_l+brakepre_dem;
    brapre_out_r=bra_pre_r+brakepre_dem;
    mode=14;
elseif flag_lf==0 && flag_lr==1 &&flag_rf==1 && flag_rr==1 %左前不滑转
    trq_out_rf=trq_pid_rf;
    trq_out_rr=trq_pid_rr;
    trq_out_lr=trq_pid_lr;
    trq_out_lf=trq_dem_lf+(trq_dem_lr-trq_out_lr)-(trq_dem_rf+trq_dem_rr-trq_out_rf-trq_out_rr);
    brapre_out_l=bra_pre_l+brakepre_dem;
    brapre_out_r=bra_pre_r+brakepre_dem;
    mode=15;
else
    %     flag_lf==1 && flag_lr==1 &&flag_rf==1 && flag_rr==1 %4电机均滑转======================================================================4电机均滑转
    trqcha=(trq_pid_lf+trq_pid_lr)-(trq_pid_rf+trq_pid_rr);
    if trqcha>0
        trq_out_rf=trq_pid_rf;
        trq_out_rr=trq_pid_rr;
        trq_out_lf=trq_pid_lf-(trq_pid_lf/(trq_pid_lf+trq_pid_lr))*trqcha;
        trq_out_lr=trq_pid_lr-(trq_pid_lr/(trq_pid_lf+trq_pid_lr))*trqcha;
    else
        trq_out_lf=trq_pid_lf;
        trq_out_lr=trq_pid_lr;
        trq_out_rf=trq_pid_rf+(trq_pid_rf/(trq_pid_rf+trq_pid_rr))*trqcha;
        trq_out_rr=trq_pid_rr+(trq_pid_rr/(trq_pid_rf+trq_pid_rr))*trqcha;
    end
    brapre_out_l=bra_pre_l+brakepre_dem;
    brapre_out_r=bra_pre_r+brakepre_dem;
    mode=16;
end
trq_out_lf=max(0,trq_out_lf);
trq_out_lr=max(0,trq_out_lr);
trq_out_rf=max(0,trq_out_rf);
trq_out_rr=max(0,trq_out_rr);
brapre_out_l=brapre_out_l;
brapre_out_r=brapre_out_r;
end

== system DDCU_wxt_v02_forA_OpenLoop/MainControl/mode_control/neutral/neutral ==
  Signals : Inport
  Bus Selector : BusSelector  OutputSignals=YaoKong.brake_dem
  Constant : Constant  Value=0
  Gain : Gain  Gain=1/2
  HeartBeat : MATLAB Function  TreatAsAtomicUnit=on
  HeartBeat1 : MATLAB Function  TreatAsAtomicUnit=on
  Memory : Memory  InheritSampleTime=on
  Memory1 : Memory  InheritSampleTime=on
  Mux : Mux  Inputs=8
  Mux1 : Mux  Inputs=8
  Mux2 : Mux  Inputs=7
  Mux3 : Mux  Inputs=7
  SpdLim_dem{,1..3} (4 alike) : Constant  Value=spdmax
  SpdSet_dem{,1..3} (4 alike) : Constant
  Terminator : Terminator
  TrqLim_dem{,1..3} (4 alike) : Constant
  TrqSet_dem{,1..3} (4 alike) : Constant  Value=0
  mot_drive : Constant
  mot_drive1 : Constant  Value=2
  mot_drive2 : Constant
  mot_drive3 : Constant  Value=2
  mot_enable{,1..3} (4 alike) : Constant  Value=2
  mot_mode{,1..3} (4 alike) : Constant
  mot_lf : Outport
  mot_lr : Outport  Port=2
  mot_rf : Outport  Port=3
  mot_rr : Outport  Port=4
  bra_pre_l : Outport  Port=5
  bra_pre_r : Outport  Port=6
  wires:
  mot_drive/1 -> Mux/3
  mot_mode/1 -> Mux/2
  TrqSet_dem/1 -> Mux/4
  mot_enable/1 -> Mux/1
  SpdSet_dem/1 -> Mux/5
  Mux/1 -> mot_lf/1
  Signals/1 -> Bus Selector/1
  Bus Selector/1 -> Gain/1  "<brake_dem>"
  TrqLim_dem/1 -> Mux/6
  HeartBeat/1(life) -> Mux/8, Memory/1
  Memory/1 -> HeartBeat/1(life_pre)
  SpdLim_dem/1 -> Mux/7
  mot_drive1/1 -> Mux2/3
  mot_mode2/1 -> Mux2/2
  TrqSet_dem1/1 -> Mux2/4
  mot_enable2/1 -> Mux2/1
  SpdSet_dem1/1 -> Mux2/5
  Mux2/1 -> mot_rf/1
  TrqLim_dem1/1 -> Mux2/6
  SpdLim_dem1/1 -> Mux2/7
  mot_drive2/1 -> Mux1/3
  mot_mode1/1 -> Mux1/2
  TrqSet_dem2/1 -> Mux1/4
  mot_enable1/1 -> Mux1/1
  SpdSet_dem2/1 -> Mux1/5
  Mux1/1 -> mot_lr/1
  TrqLim_dem2/1 -> Mux1/6
  HeartBeat1/1(life) -> Mux1/8, Memory1/1
  Memory1/1 -> HeartBeat1/1(life_pre)
  SpdLim_dem2/1 -> Mux1/7
  mot_drive3/1 -> Mux3/3
  mot_mode3/1 -> Mux3/2
  TrqSet_dem3/1 -> Mux3/4
  mot_enable3/1 -> Mux3/1
  SpdSet_dem3/1 -> Mux3/5
  Mux3/1 -> mot_rr/1
  TrqLim_dem3/1 -> Mux3/6
  SpdLim_dem3/1 -> Mux3/7
  Gain/1 -> Terminator/1
  Constant/1 -> bra_pre_r/1, bra_pre_l/1

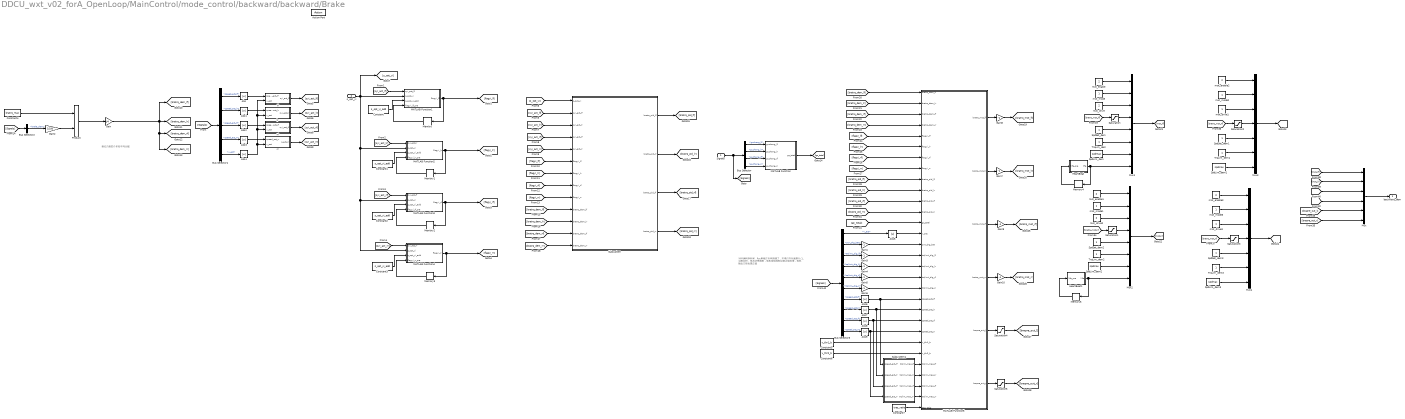
== system DDCU_wxt_v02_forA_OpenLoop/MainControl/mode_control/backward/backward/Brake ==
  note: 制动力矩四个车轮平均分配
  note: 当时编程序时候，fcn里面正负号搞错了，不得已在外面乘以-1，
      | 当制动时，电池功率限制，电机扭矩限制当做正值处理，电机
      | 输出力矩也是正值
  Signals : Inport
  s_opt_yi : Inport  Port=2
  Action Port : ActionPort  ActionType=case
  Abs{,1..9} (10 alike) : Abs
  Bus Selector : BusSelector  OutputSignals=DriveMotor.guzhang_lf,DriveMotor.guzhang_lr,DriveMotor.guzhang_rf,DriveMotor.guzhang_rr
  Bus Selector1 : BusSelector  OutputSignals=DriveMotor.speed_act_lf,DriveMotor.speed_act_lr,DriveMotor.speed_act_rf,DriveMotor.speed_act_rr,IMU.v_act
  Bus Selector2 : BusSelector  OutputSignals=YaoKong.brake_dem
  Bus Selector3 : BusSelector  OutputSignals=IMU.v_act,Bat.pwr_chg_bat,DriveMotor.trqlimL_dig_lf,DriveMotor.trqlimL_dig_lr,DriveMotor.trqlimL_dig_rf,DriveMotor.trqlimL_dig_rr,DriveMotor.speed_act_lf,DriveMotor.speed_act_lr,DriveMotor.speed_act_rf,DriveMotor.speed_act_rr
  Constant{,1..3} (4 alike) : Constant  Value=s_opt_yi_add
  Constant4 : Constant  Value=bratrq_max
  Constant5 : Constant  Value=v_thr1_b
  Constant6 : Constant  Value=v_thr2_b
  Constant7 : Constant  Value=tras_ratio
  Gain : Gain  Gain=1/4
  Gain{1,3..10} (9 alike) : Gain  Gain=-1
  Gain2 : Gain  Gain=1/100
  HeartBeat : MATLAB Function  TreatAsAtomicUnit=on
  HeartBeat1 : MATLAB Function  TreatAsAtomicUnit=on
  MATLAB Function : MATLAB Function  TreatAsAtomicUnit=on
  MATLAB Function1 : MATLAB Function  TreatAsAtomicUnit=on
  MATLAB Function2 : MATLAB Function  TreatAsAtomicUnit=on
  MATLAB Function3 : MATLAB Function  TreatAsAtomicUnit=on
  MATLAB Function4 : MATLAB Function  TreatAsAtomicUnit=on
  MATLAB Function5 : MATLAB Function  TreatAsAtomicUnit=on
  Memory{,1..5} (6 alike) : Memory  InheritSampleTime=on
  Mux : Mux  Inputs=6
  Mux1 : Mux  Inputs=8
  Mux2 : Mux  Inputs=8
  Mux3 : Mux  Inputs=7
  Mux4 : Mux  Inputs=7
  Product : Product
  Saturation{,1..3} (4 alike) : Saturate  UpperLimit=0  LowerLimit=-trqmax
  Saturation4 : Saturate  UpperLimit=premax  LowerLimit=0
  Saturation5 : Saturate  UpperLimit=premax  LowerLimit=0
  SpdLim_dem{,1..3} (4 alike) : Constant  Value=spdmax
  SpdSet_dem{,1..3} (4 alike) : Constant
  Subsystem : Subsystem
  Subsystem1 : Subsystem
  TrqLim_dem{,1..3} (4 alike) : Constant
  lf : Subsystem
  lr : Subsystem
  mot_drive : Constant  Value=2
  mot_drive1 : Constant
  mot_drive2 : Constant  Value=2
  mot_drive3 : Constant
  mot_enable{,1..3} (4 alike) : Constant  Value=2
  mot_mode{,1..3} (4 alike) : Constant
  rf : Subsystem
  rr : Subsystem
  backward_dem : Outport
  wires:
  Saturation5/1 -> [brapre_out_r]
  Saturation4/1 -> [brapre_out_l]
  Saturation3/1 -> Mux4/4
  Saturation2/1 -> Mux3/4
  Saturation1/1 -> Mux2/4
  Saturation/1 -> Mux1/4
  Gain10/1 -> [bratrq_mot_rr]
  Gain9/1 -> [bratrq_mot_rf]
  Gain7/1 -> [bratrq_mot_lr]
  Gain8/1 -> [bratrq_mot_lf]
  [bratrq_mot_lf] -> Saturation/1
  Constant5/1 -> MATLAB Function5/24(v_thr1_b)
  Subsystem1/1(trqlim_map_lf) -> MATLAB Function5/26(trqlim_map_lf)
  Subsystem1/2(trqlim_map_lr) -> MATLAB Function5/27(trqlim_map_lr)
  Subsystem1/3(trqlim_map_rf) -> MATLAB Function5/28(trqlim_map_rf)
  Subsystem1/4(trqlim_map_rr) -> MATLAB Function5/29(trqlim_map_rr)
  [gz_total] -> MATLAB Function5/13(gz_total)
  [bratrq_pid_rr] -> MATLAB Function5/12(bratrq_pid_rr)
  [bratrq_pid_rf] -> MATLAB Function5/11(bratrq_pid_rf)
  [bratrq_pid_lr] -> MATLAB Function5/10(bratrq_pid_lr)
  [bratrq_pid_lf] -> MATLAB Function5/9(bratrq_pid_lf)
  [flagyi_rr] -> MATLAB Function5/8(flagyi_rr)
  [flagyi_rf] -> MATLAB Function5/7(flagyi_rf)
  [flagyi_lr] -> MATLAB Function5/6(flagyi_lr)
  [flagyi_lf] -> MATLAB Function5/5(flagyi_lf)
  [bratrq_dem_rr] -> MATLAB Function5/4(bratrq_dem_rr)
  [bratrq_dem_lf] -> MATLAB Function5/1(bratrq_dem_lf)
  [bratrq_dem_rf] -> MATLAB Function5/3(bratrq_dem_rf)
  [bratrq_dem_lr] -> MATLAB Function5/2(bratrq_dem_lr)
  Gain6/1 -> MATLAB Function5/19(trqlimL_dig_rr)
  Gain5/1 -> MATLAB Function5/18(trqlimL_dig_rf)
  Gain4/1 -> MATLAB Function5/17(trqlimL_dig_lr)
  Gain3/1 -> MATLAB Function5/16(trqlimL_dig_lf)
  Gain1/1 -> MATLAB Function5/15(pwr_chg_bat)
  Constant6/1 -> MATLAB Function5/25(v_thr2_b)
  Product/1 -> Gain/1
  Bus Selector2/1 -> Gain2/1  "<brake_dem>"
  Gain2/1 -> Product/2
  Constant4/1 -> Product/1
  Bus Selector3/10 -> Abs9/1  "<speed_act_rr>"
  Bus Selector3/9 -> Abs8/1  "<speed_act_rf>"
  Bus Selector3/8 -> Abs7/1  "<speed_act_lr>"
  Bus Selector3/7 -> Abs6/1  "<speed_act_lf>"
  Bus Selector3/6 -> Gain6/1  "<trqlimL_dig_rr>"
  Bus Selector3/5 -> Gain5/1  "<trqlimL_dig_rf>"
  Bus Selector3/4 -> Gain4/1  "<trqlimL_dig_lr>"
  Bus Selector3/3 -> Gain3/1  "<trqlimL_dig_lf>"
  Bus Selector3/1 -> Abs5/1  "<v_act>"
  Bus Selector3/2 -> Gain1/1  "<pwr_chg_bat>"
  [Signals] -> Bus Selector3/1
  MATLAB Function5/6(brapre_out_r) -> Saturation5/1
  MATLAB Function5/5(brapre_out_l) -> Saturation4/1
  MATLAB Function5/4(bratrq_mot_rr) -> Gain10/1
  MATLAB Function5/2(bratrq_mot_lr) -> Gain7/1
  MATLAB Function5/3(bratrq_mot_rf) -> Gain9/1
  MATLAB Function5/1(bratrq_mot_lf) -> Gain8/1
  [brapre_out_r] -> Mux/6
  [brapre_out_l] -> Mux/5
  [mot_rr] -> Mux/4
  [mot_rf] -> Mux/3
  [mot_lr] -> Mux/2
  [mot_lf] -> Mux/1
  mot_drive/1 -> Mux1/3
  mot_mode/1 -> Mux1/2
  mot_enable/1 -> Mux1/1
  SpdSet_dem/1 -> Mux1/5
  Mux1/1 -> [mot_lf]
  TrqLim_dem/1 -> Mux1/6
  HeartBeat/1(life) -> Mux1/8, Memory4/1
  Memory4/1 -> HeartBeat/1(life_pre)
  SpdLim_dem/1 -> Mux1/7
  mot_drive1/1 -> Mux3/3
  mot_mode2/1 -> Mux3/2
  [bratrq_mot_rf] -> Saturation2/1
  mot_enable2/1 -> Mux3/1
  SpdSet_dem1/1 -> Mux3/5
  Mux3/1 -> [mot_rf]
  TrqLim_dem1/1 -> Mux3/6
  SpdLim_dem1/1 -> Mux3/7
  mot_drive2/1 -> Mux2/3
  mot_mode1/1 -> Mux2/2
  [bratrq_mot_lr] -> Saturation1/1
  mot_enable1/1 -> Mux2/1
  SpdSet_dem2/1 -> Mux2/5
  Mux2/1 -> [mot_lr]
  TrqLim_dem2/1 -> Mux2/6
  HeartBeat1/1(life) -> Mux2/8, Memory5/1
  Memory5/1 -> HeartBeat1/1(life_pre)
  SpdLim_dem2/1 -> Mux2/7
  mot_drive3/1 -> Mux4/3
  mot_mode3/1 -> Mux4/2
  [bratrq_mot_rr] -> Saturation3/1
  mot_enable3/1 -> Mux4/1
  SpdSet_dem3/1 -> Mux4/5
  Mux4/1 -> [mot_rr]
  TrqLim_dem3/1 -> Mux4/6
  SpdLim_dem3/1 -> Mux4/7
  Mux/1 -> backward_dem/1
  Subsystem/4(bratrq_pid_rr) -> [bratrq_pid_rr]
  Subsystem/1(bratrq_pid_lf) -> [bratrq_pid_lf]
  Subsystem/3(bratrq_pid_rf) -> [bratrq_pid_rf]
  Subsystem/2(bratrq_pid_lr) -> [bratrq_pid_lr]
  [bratrq_dem_rr] -> Subsystem/13(bratrq_dem_rr)
  [bratrq_dem_rf] -> Subsystem/12(bratrq_dem_rf)
  [bratrq_dem_lr] -> Subsystem/11(bratrq_dem_lr)
  [bratrq_dem_lf] -> Subsystem/10(bratrq_dem_lf)
  Gain/1 -> [bratrq_dem_lf], [bratrq_dem_rf], [bratrq_dem_rr], [bratrq_dem_lr]
  [Signals] -> Bus Selector2/1
  [flagyi_rr] -> Subsystem/9(flagyi_rr)
  [flagyi_lr] -> Subsystem/7(flagyi_lr)
  [flagyi_lf] -> Subsystem/6(flagyi_lf)
  [flagyi_rf] -> Subsystem/8(flagyi_rf)
  [syi_act_rr] -> Subsystem/5(syi_act_rr)
  [syi_act_rf] -> Subsystem/4(syi_act_rf)
  [syi_act_lr] -> Subsystem/3(syi_act_lr)
  [syi_act_lf] -> Subsystem/2(syi_act_lf)
  [s_opt_yi] -> Subsystem/1(s_opt_yi)
  [syi_act_rr] -> MATLAB Function4/1(syi_act_rr)
  [syi_act_rf] -> MATLAB Function3/1(syi_act_rf)
  [syi_act_lr] -> MATLAB Function2/1(syi_act_lr)
  [syi_act_lf] -> MATLAB Function1/1(syi_act_lf)
  rr/1(s_act_rr) -> [syi_act_rr]
  rf/1(syi_act_rf) -> [syi_act_rf]
  lf/1(syi_act_lf) -> [syi_act_lf]
  lr/1(syi_act_lr) -> [syi_act_lr]
  MATLAB Function1/1(flagyi_lf) -> Memory/1, [flagyi_lf]
  Memory/1 -> MATLAB Function1/4(flagyi_lf_pre)
  Constant/1 -> MATLAB Function1/3(s_opt_yi_add)
  MATLAB Function2/1(flagyi_lr) -> [flagyi_lr], Memory1/1
  Memory1/1 -> MATLAB Function2/4(flagyi_lr_pre)
  Constant1/1 -> MATLAB Function2/3(s_opt_yi_add)
  MATLAB Function3/1(flagyi_rf) -> Memory2/1, [flagyi_rf]
  Memory2/1 -> MATLAB Function3/4(flagyi_rf_pre)
  Constant2/1 -> MATLAB Function3/3(s_opt_yi_add)
  s_opt_yi/1 -> [s_opt_yi], MATLAB Function1/2(s_opt_yi), MATLAB Function4/2(s_opt_yi), MATLAB Function3/2(s_opt_yi), MATLAB Function2/2(s_opt_yi)
  MATLAB Function4/1(flagyi_rr) -> [flagyi_rr], Memory3/1
  Memory3/1 -> MATLAB Function4/4(flagyi_rr_pre)
  Constant3/1 -> MATLAB Function4/3(s_opt_yi_add)
  Bus Selector1/5 -> Abs4/1  "<v_act>"
  Bus Selector1/4 -> Abs3/1  "<speed_act_rr>"
  Bus Selector1/3 -> Abs2/1  "<speed_act_rf>"
  Bus Selector1/2 -> Abs1/1  "<speed_act_lr>"
  Bus Selector1/1 -> Abs/1  "<speed_act_lf>"
  [Signals] -> Bus Selector1/1
  MATLAB Function/1(gz_total) -> [gz_total]
  Bus Selector/1 -> MATLAB Function/1(guzhang_lf)  "<guzhang_lf>"
  Bus Selector/2 -> MATLAB Function/2(guzhang_lr)  "<guzhang_lr>"
  Bus Selector/4 -> MATLAB Function/4(guzhang_rr)  "<guzhang_rr>"
  Bus Selector/3 -> MATLAB Function/3(guzhang_rf)  "<guzhang_rf>"
  Signals/1 -> Bus Selector/1, [Signals]
  Abs/1 -> lf/1(speed_act_lf)
  Abs1/1 -> lr/1(speed_act_lr)
  Abs2/1 -> rf/1(speed_act_rf)
  Abs3/1 -> rr/1(speed_act_rr)
  Abs4/1 -> lf/2(v_act), lr/2(v_act), rf/2(v_act), rr/2(v_act)
  Abs5/1 -> MATLAB Function5/14(v_act)
  Abs6/1 -> MATLAB Function5/20(speed_act_lf), Subsystem1/1(speed_act_lf)
  Abs7/1 -> MATLAB Function5/21(speed_act_lr), Subsystem1/2(speed_act_lr)
  Abs8/1 -> MATLAB Function5/22(speed_act_rf), Subsystem1/3(speed_act_rf)
  Abs9/1 -> MATLAB Function5/23(speed_act_rr), Subsystem1/4(speed_act_rr)
  Constant7/1 -> MATLAB Function5/30(tras_ratio)
